simulink model "TENNIS_Ball"  (Simulink 7.4)
settings: Solver=ode4  StartTime=0.0  StopTime=1.5  FixedStep=.01  RelTol=1e-7
values from neighbouring files (symbols this model uses):
  eta = 1    [BallPosition_2D_ODE.m]    (also in BallPosition_3D_ODE.m = -1; RUN_all.m = ETA(ii); objectivefun.m; simulateTrajectory.m)
libraries: simulink x3
settings Model: Creator=SLE  LastModifiedBy=David
settings DataIOCC: Decimation=4  LimitDataPoints=off  SignalLogging=off  SaveTime=off
settings RTWCC: GenCodeOnly=on  GenerateReport=on  TLCDebug=on  TLCAssert=on  RTWUseSimCustomCode=on  LaunchReport=on  TargetLang=C++
settings CodeAppCC: ForceParamTrailComments=on  UseSimReservedNames=on

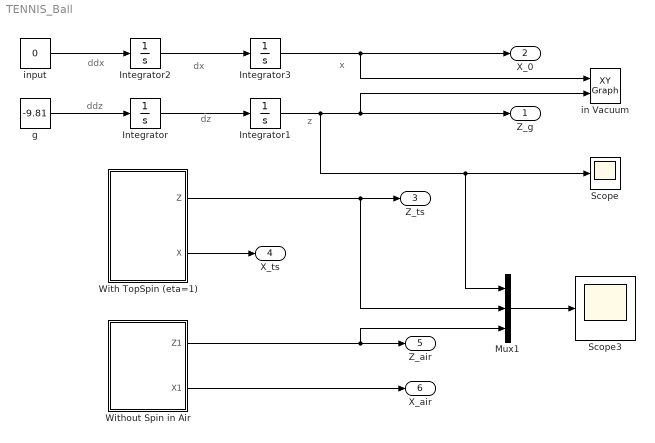
== system TENNIS_Ball ==
  note: dx
  note: x
  note: dz
  note: ddz
  note: z
  note: ddx
  Integrator : Integrator  InitialCondition=25*sin(15*pi/180)
  Integrator1 : Integrator  InitialCondition=1
  Integrator2 : Integrator  InitialCondition=25*cos(15*pi/180)
  Integrator3 : Integrator
  Mux1 : Mux  Inputs=3
  Scope : Scope
      settings: YMin=0  YMax=3.35  DataFormat=Array
  Scope3 : Scope
      settings: TickLabels=on  YMin=0  YMax=3.5  SaveName=ScopeData4  DataFormat=Array
  With TopSpin (eta=1) : Subsystem
  Without Spin in Air : Subsystem
  g : Constant  Value=-9.81
  in Vacuum : simulink/Sinks/XY Graph  SystemSampleTime=-1  xmin=0  xmax=36  ymin=-.1  ymax=3.35  st=-1
  input : Constant  Value=0
  Z_g : Outport
  X_0 : Outport  Port=2
  Z_ts : Outport  Port=3
  X_ts : Outport  Port=4
  Z_air : Outport  Port=5
  X_air : Outport  Port=6
  wires:
  Integrator/1 -> Integrator1/1
  Integrator1/1 -> Z_g/1, in Vacuum/2, Scope/1, Mux1/1
  Integrator2/1 -> Integrator3/1
  Integrator3/1 -> X_0/1, in Vacuum/1
  g/1 -> Integrator/1
  input/1 -> Integrator2/1
  With TopSpin (eta=1)/1(Z) -> Z_ts/1, Mux1/2
  With TopSpin (eta=1)/2(X) -> X_ts/1
  Without Spin in Air/1(Z1) -> Z_air/1, Mux1/3
  Without Spin in Air/2(X1) -> X_air/1
  Mux1/1 -> Scope3/1

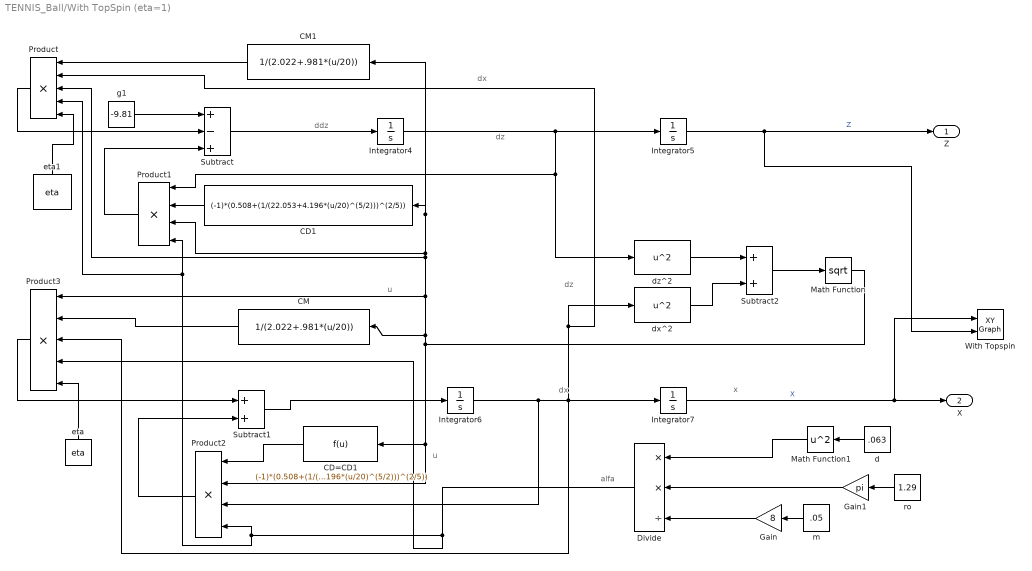
== system TENNIS_Ball/With TopSpin (eta=1) ==
  note: dx
  note: dz
  note: dx
  note: u
  note: u
  note: x
  note: dz
  note: ddz
  note: alfa
  CD1 : Fcn  Expr=(-1)*(0.508+(1/(22.053+4.196*(u/20)^(5/2)))^(2/5))
  CD=CD1 : Fcn  Expr=(-1)*(0.508+(1/(22.053+4.196*(u/20)^(5/2)))^(2/5))
  CM : Fcn  Expr=1/(2.022+.981*(u/20))
  CM1 : Fcn  Expr=1/(2.022+.981*(u/20))
  Divide : Product  Inputs=**/
  Gain : Gain  Gain=8
  Gain1 : Gain  Gain=pi
  Integrator4 : Integrator  InitialCondition=25*sin(15*pi/180)
  Integrator5 : Integrator  InitialCondition=1
  Integrator6 : Integrator  InitialCondition=25*cos(15*pi/180)
  Integrator7 : Integrator
  Math Function : Math  Operator=sqrt  SaturateOnIntegerOverflow=on
  Math Function1 : Math  Operator=square  SaturateOnIntegerOverflow=on
  Product : Product  Inputs=5  RndMeth=Zero
  Product1 : Product  Inputs=4  RndMeth=Zero
  Product2 : Product  Inputs=4  RndMeth=Zero
  Product3 : Product  Inputs=5  RndMeth=Zero
  Subtract : Sum  Inputs=+-+
  Subtract1 : Sum
  Subtract2 : Sum
  With Topspin : simulink/Sinks/XY Graph  SystemSampleTime=-1  xmin=0  xmax=36  ymin=-.1  ymax=3.35  st=-1
  d : Constant  Value=.063
  dx^2 : Fcn  Expr=u^2
  dz^2 : Fcn  Expr=u^2
  eta : Constant  Value=eta
  eta1 : Constant  Value=eta
  g1 : Constant  Value=-9.81
  m : Constant  Value=.05
  ro : Constant  Value=1.29
  Z : Outport
  X : Outport  Port=2
  wires:
  Integrator4/1 -> Integrator5/1, dz^2/1, Product1/1
  Integrator5/1 -> Z/1, With Topspin/2  "Z"
  Integrator6/1 -> Integrator7/1, Product3/3, dx^2/1, Product/2, Product2/3
  Integrator7/1 -> X/1, With Topspin/1  "X"
  Subtract/1 -> Integrator4/1
  Subtract1/1 -> Integrator6/1
  Product2/1 -> Subtract1/2
  CM/1 -> Product3/2
  Product3/1 -> Subtract1/1
  g1/1 -> Subtract/1
  CD1/1 -> Product1/2
  Product1/1 -> Subtract/3
  CM1/1 -> Product/1
  Product/1 -> Subtract/2
  dz^2/1 -> Subtract2/1
  dx^2/1 -> Subtract2/2
  Subtract2/1 -> Math Function/1
  Math Function/1 -> Product1/3, CD1/1, CM1/1, Product/3, Product3/1, CM/1, Product2/2, CD=CD1/1
  Divide/1 -> Product3/4, Product2/4, Product1/4, Product/4
  CD=CD1/1 -> Product2/1
  Gain/1 -> Divide/3
  Gain1/1 -> Divide/2
  Math Function1/1 -> Divide/1
  ro/1 -> Gain1/1
  m/1 -> Gain/1
  d/1 -> Math Function1/1
  eta1/1 -> Product/5
  eta/1 -> Product3/5

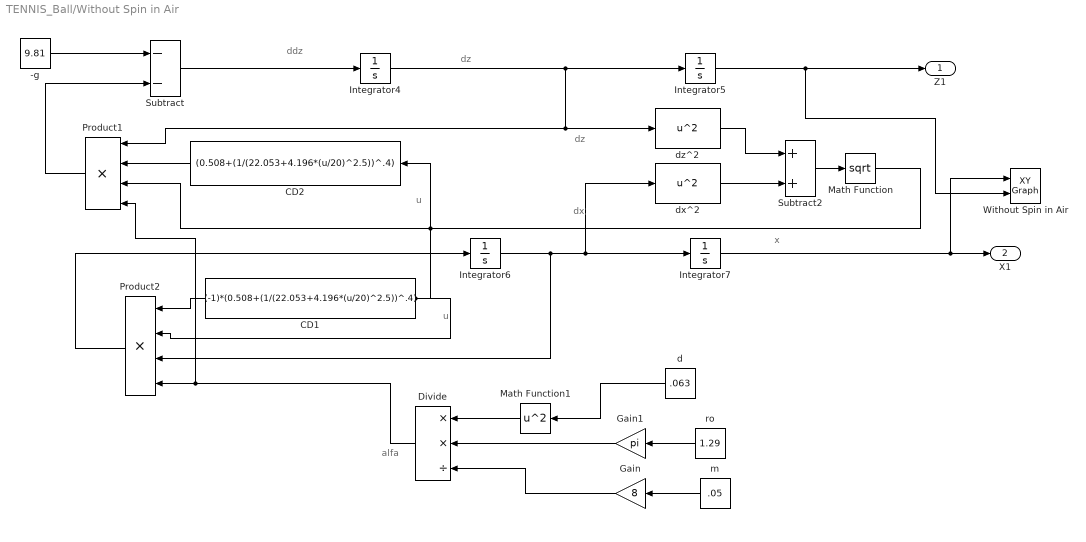
== system TENNIS_Ball/Without Spin in Air ==
  note: dz
  note: dx
  note: u
  note: u
  note: x
  note: dz
  note: ddz
  note: alfa
  -g : Constant  Value=9.81
  CD1 : Fcn  Expr=(-1)*(0.508+(1/(22.053+4.196*(u/20)^2.5))^.4)
  CD2 : Fcn  Expr=(0.508+(1/(22.053+4.196*(u/20)^2.5))^.4)
  Divide : Product  Inputs=**/
  Gain : Gain  Gain=8
  Gain1 : Gain  Gain=pi
  Integrator4 : Integrator  InitialCondition=25*sin(15*pi/180)
  Integrator5 : Integrator  InitialCondition=1
  Integrator6 : Integrator  InitialCondition=25*cos(15*pi/180)
  Integrator7 : Integrator
  Math Function : Math  Operator=sqrt  OutDataType=fixdt(1, 16)  OutScaling=2^0  SaturateOnIntegerOverflow=on
  Math Function1 : Math  Operator=square  SaturateOnIntegerOverflow=on
  Product1 : Product  Inputs=4  RndMeth=Zero
  Product2 : Product  Inputs=4  RndMeth=Zero
  Subtract : Sum  Inputs=--
  Subtract2 : Sum
  Without Spin in Air : simulink/Sinks/XY Graph  SystemSampleTime=-1  xmin=0  xmax=36  ymin=-.1  ymax=3.35  st=-1
  d : Constant  Value=.063
  dx^2 : Fcn  Expr=u^2
  dz^2 : Fcn  Expr=u^2
  m : Constant  Value=.05
  ro : Constant  Value=1.29
  Z1 : Outport
  X1 : Outport  Port=2
  wires:
  Integrator4/1 -> Integrator5/1, Product1/1, dz^2/1
  Integrator5/1 -> Z1/1, Without Spin in Air/2
  Integrator6/1 -> Integrator7/1, dx^2/1, Product2/3
  Integrator7/1 -> X1/1, Without Spin in Air/1
  Subtract/1 -> Integrator4/1
  Product2/1 -> Integrator6/1
  -g/1 -> Subtract/1
  CD2/1 -> Product1/2
  Product1/1 -> Subtract/2
  dz^2/1 -> Subtract2/1
  dx^2/1 -> Subtract2/2
  Subtract2/1 -> Math Function/1
  Math Function/1 -> Product1/3, Product2/2, CD1/1, CD2/1
  d/1 -> Math Function1/1
  ro/1 -> Gain1/1
  Math Function1/1 -> Divide/1
  Gain1/1 -> Divide/2
  Divide/1 -> Product2/4, Product1/4
  CD1/1 -> Product2/1
  m/1 -> Gain/1
  Gain/1 -> Divide/3
